simulink library "Robust_MPC_LibraryMDLversion"  (Simulink 8.1)
settings: Solver=ode45  StartTime=0.0  StopTime=10.0  RelTol=1e-3
undefined symbols (not defined in the file or in its folder): sol_x_mp
undefined symbols (not defined in the file): add_usys_d, TTR_RobustMPC
settings Model: Creator=Kostas  LastModifiedBy=Kostas

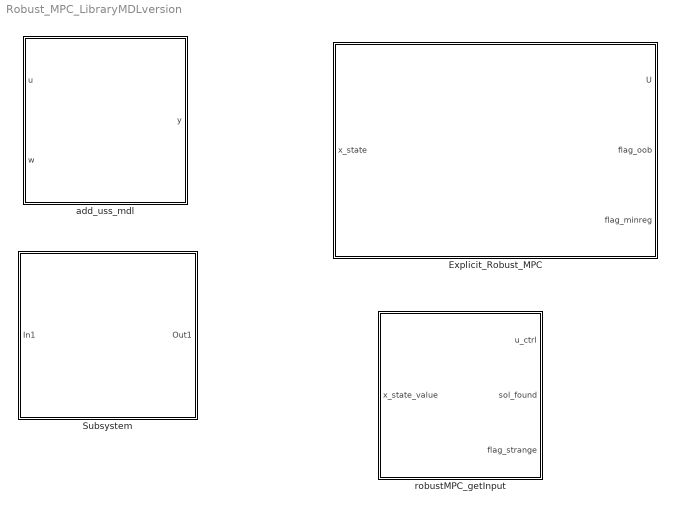
== system Robust_MPC_LibraryMDLversion ==
  Explicit_Robust_MPC : Subsystem  mask{H=TTR_RobustMPC.Zdir.Explicit.H, K=TTR_RobustMPC.Zdir.Explicit.K, F=TTR_RobustMPC.Zdir.Explicit.F, G=TTR_RobustMPC.Zdir.Explicit.G, Nc=TTR_RobustMPC.Zdir.Explicit.Nc, Nx=TTR_RobustMPC.Zdir.Explicit.Nx, Hi_init=zeros(100,TTR_RobustMPC.Zdir.Explicit.Nx), Ki_init=0}
      mask prompts: H "Explicit Robust MPC {H}"; K "Explicit Robust MPC {K}"; F "Explicit Robust MPC {F}"; G "Explicit Robust MPC {G}"; Nc "Explicit Robust MPC {Nc}"; Nx "Explicit Robust MPC {Nx}"; Hi_init "Explicit Robust MPC {Hinit}"; Ki_init "Explicit Robust MPC {Kinit}"
      mask Display:
      | port_label('input',1,'x_state');
      | port_label('output',1,'U');
      | port_label('output',2,'flag_oob');
      | disp('Explicit Robust MPC')
      | plot([10 20 30 40],[10 20 20 25])
  Subsystem : Subsystem
  add_uss_mdl : Subsystem  mask{add_usys_d_struct=add_usys_d}
      mask prompts: add_usys_d_struct "Provide Additive Uncertainty Structure"
  robustMPC_getInput : Subsystem

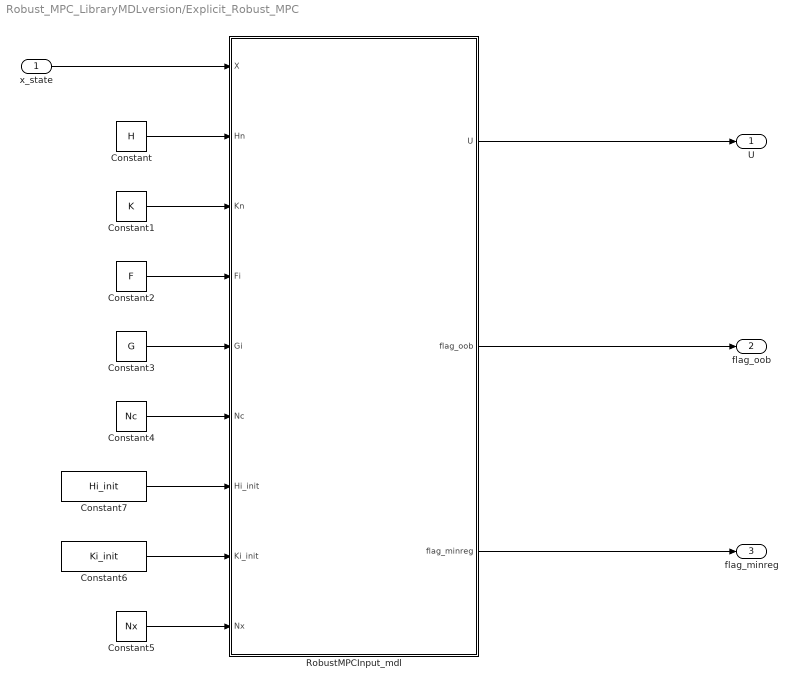
== system Robust_MPC_LibraryMDLversion/Explicit_Robust_MPC ==
  x_state : Inport
  Constant : Constant  Value=H
  Constant1 : Constant  Value=K
  Constant2 : Constant  Value=F
  Constant3 : Constant  Value=G
  Constant4 : Constant  Value=Nc
  Constant5 : Constant  Value=Nx
  Constant6 : Constant  Value=Ki_init
  Constant7 : Constant  Value=Hi_init
  RobustMPCInput_mdl : MATLAB Function  TreatAsAtomicUnit=on
  U : Outport
  flag_oob : Outport  Port=2
  flag_minreg : Outport  Port=3
  wires:
  Constant/1 -> RobustMPCInput_mdl/2(Hn)
  Constant1/1 -> RobustMPCInput_mdl/3(Kn)
  Constant2/1 -> RobustMPCInput_mdl/4(Fi)
  Constant3/1 -> RobustMPCInput_mdl/5(Gi)
  Constant4/1 -> RobustMPCInput_mdl/6(Nc)
  Constant5/1 -> RobustMPCInput_mdl/9(Nx)
  Constant7/1 -> RobustMPCInput_mdl/7(Hi_init)
  x_state/1 -> RobustMPCInput_mdl/1(X)
  RobustMPCInput_mdl/1(U) -> U/1
  RobustMPCInput_mdl/2(flag_oob) -> flag_oob/1
  Constant6/1 -> RobustMPCInput_mdl/8(Ki_init)
  RobustMPCInput_mdl/3(flag_minreg) -> flag_minreg/1

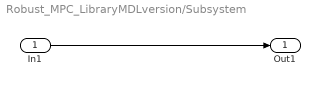
== system Robust_MPC_LibraryMDLversion/Subsystem ==
  In1 : Inport
  Out1 : Outport
  wires:
  In1/1 -> Out1/1

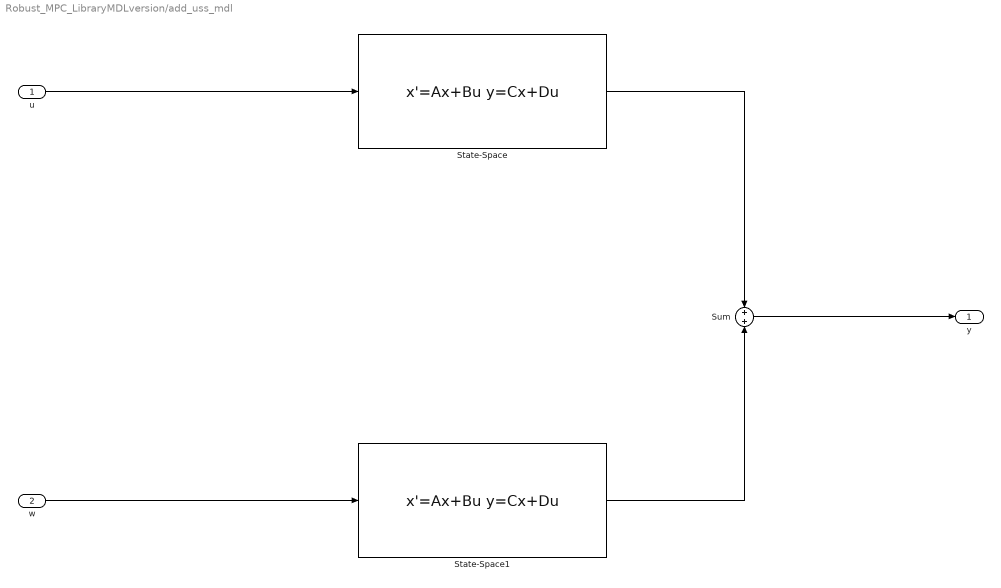
== system Robust_MPC_LibraryMDLversion/add_uss_mdl ==
  u : Inport
  w : Inport  Port=2
  State-Space : StateSpace  A=add_usys_d_struct.continuous.matrices.A  B=add_usys_d_struct.continuous.matrices.B  C=add_usys_d_struct.continuous.matrices.C  D=add_usys_d_struct.continuous.matrices.D
  State-Space1 : StateSpace  A=add_usys_d_struct.continuous.matrices.A  B=add_usys_d_struct.continuous.matrices.E  C=add_usys_d_struct.continuous.matrices.C  D=add_usys_d_struct.continuous.matrices.D
  Sum : Sum  Inputs=+|+
  y : Outport
  wires:
  u/1 -> State-Space/1
  w/1 -> State-Space1/1
  State-Space/1 -> Sum/1
  State-Space1/1 -> Sum/2
  Sum/1 -> y/1

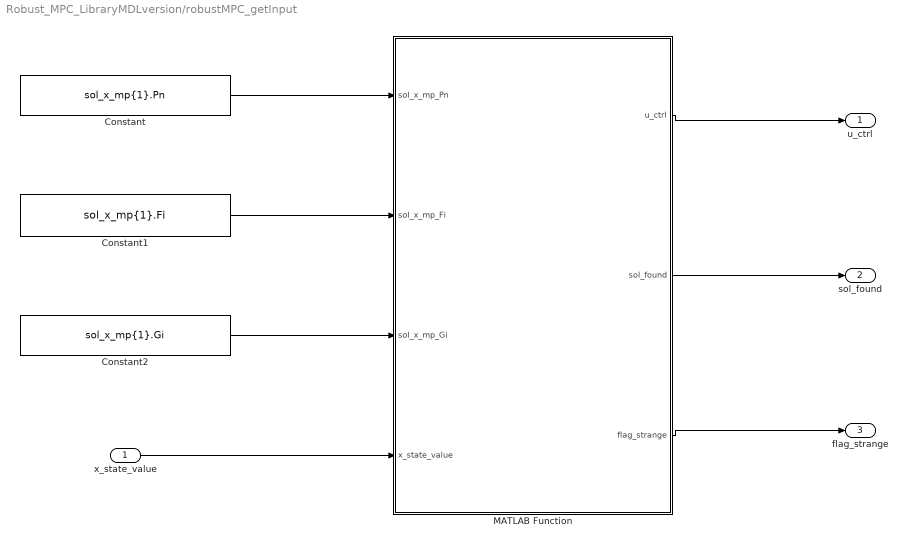
== system Robust_MPC_LibraryMDLversion/robustMPC_getInput ==
  x_state_value : Inport
  Constant : Constant  Value=sol_x_mp{1}.Pn
  Constant1 : Constant  Value=sol_x_mp{1}.Fi
  Constant2 : Constant  Value=sol_x_mp{1}.Gi
  MATLAB Function : MATLAB Function  TreatAsAtomicUnit=on
  u_ctrl : Outport
  sol_found : Outport  Port=2
  flag_strange : Outport  Port=3
  wires:
  Constant/1 -> MATLAB Function/1(sol_x_mp_Pn)
  Constant1/1 -> MATLAB Function/2(sol_x_mp_Fi)
  Constant2/1 -> MATLAB Function/3(sol_x_mp_Gi)
  x_state_value/1 -> MATLAB Function/4(x_state_value)
  MATLAB Function/1(u_ctrl) -> u_ctrl/1
  MATLAB Function/2(sol_found) -> sol_found/1
  MATLAB Function/3(flag_strange) -> flag_strange/1

== matlab function Explicit_Robust_MPC/RobustMPCInput_mdl ==
  data: X input double; U output double; Hn input double; Kn input double; Fi input double; Gi input double; Nc input double; Hi_init input double; Ki_init input double; Nx input double; flag_oob output double; flag_minreg output double
function[U,flag_oob,flag_minreg] =RobustMPCInput_mdl(X,Hn,Kn,Fi,Gi,Nc,Hi_init,Ki_init,Nx)
%#codegen

flag_minreg = 0; % a last resort safety flag

tolerance = 1;
nr  = size(Nc,1);
MPT_ABSTOL = 1e-8;
minreg = 0;
X = round(10000*X)/10000;

flag_oob = 0;
%maxSize = max(Nc);

Hi = Hi_init;
Ki = Ki_init;

% Find the proper region
abspos = 1;
for ireg = 1:nr
    sumViol = 0;
    isinside = 1;
    

  %  Hi(1:Nc(ireg),1:4) = Hn(abspos:(abspos+Nc(ireg)-1),1:4);
    for i = 1:Nc(ireg)
        for j = 1:Nx
            Hi(i,j) = Hn(abspos + i - 1,j);
        end
    end
    
%    Ki(1:Nc(ireg),1) = Kn(abspos:(abspos+Nc(ireg)-1),1);
    for i = 1:Nc(ireg)
        Ki(i,1) = Kn(abspos + i - 1,1);
    end
    abspos = abspos + Nc(ireg);
    
    F = Fi(ireg,:);
    G = Gi(ireg,:);
    
    nc = Nc(ireg);
    
    for ic = 1:nc
        hx = Hi(ic,:)*X;
        if ((hx - Ki(ic)) > MPT_ABSTOL)
            isinside = 0;
            sumViol = sumViol + (hx - Ki(ic));
        end
    end
    
    if (sumViol < tolerance)
        tolerance = sumViol;
        minreg = ireg;
    end
    % extract the right control law
    if (isinside == 1)
        U = F*X + G;
        return
    end
end

%   do some safety stuff because you never know...
size_F = size(F);
if ( (minreg==0) || (minreg > size_F(1) ) )
    flag_minreg = 1;
    minreg = 1;
end

F = Fi(minreg,:);
G = Gi(minreg,:);
U = F*X + G;
flag_oob = 1;
%U = U_prev;
return

== matlab function robustMPC_getInput/MATLAB Function ==
  data: sol_x_mp_Pn input double; sol_x_mp_Fi input double; sol_x_mp_Gi input double; u_ctrl output double; x_state_value input double; sol_found output double; flag_strange output double
function [u_ctrl,sol_found, flag_strange] = robustmpc_getInput(sol_x_mp_Pn, sol_x_mp_Fi,sol_x_mp_Gi,x_state_value)
%
%   get control action from the explicit robust mpc computed using YALMIP
%
%   Syntax:
%   [u_ctrl,sol_found] = robustmpc_getInput(sol_x_mp, x_state_value)
%
%   Inputs:
%   sol_x_mp        : Multiparametric Robust MPC explicit solution
%   x_state_value   : value of the state vector
%
%   Outputs:
%   u_ctrl          : control action
%   sol_found       : flag indicating whether a solution was found
%
%   Authors: Kostas Alexis (konstantinos.alexis@mavt.ethz.ch)

sol_found = 1;
[i,j] = isinside(sol_x_mp_Pn, x_state_value);

flag_strange = 0;
if(length(j)>1)
    j = j(1); % this requires further analysis
    flag_strange = 1;
end

if(isempty(j)==0)
    u_ctrl = sol_x_mp_Fi{j}*x_state_value + sol_x_mp_Gi{j};
    sol_found = 1;
else
    sol_found = 0;
    u_ctrl = NaN;
end

if(flag_strange == 1)
    u_ctrl = 0.0256;
end
end
